simulink model "majorPonepointO1"  (R2023a)
settings: Solver=VariableStepAuto  StartTime=0.0  StopTime=100  RelTol=1e-3
libraries: slpidlib x1
settings Model: Creator=rahul  LastModifiedBy=rahul

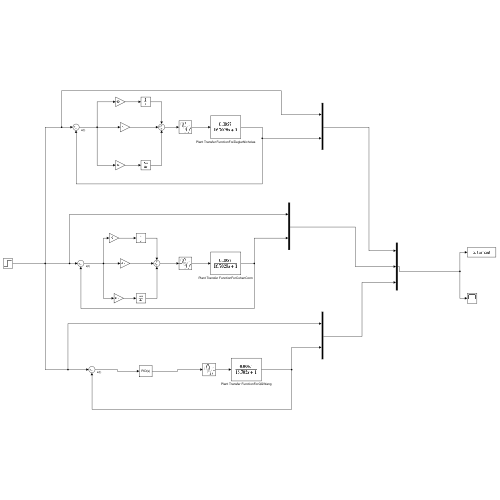
[thumbnail: Simulink's stored preview of the top-level diagram]
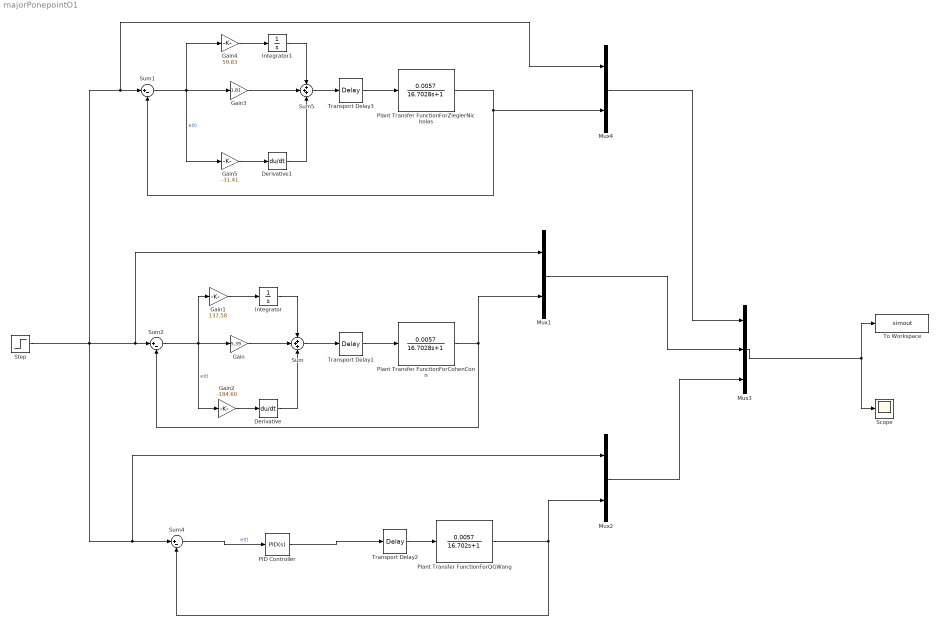
== system majorPonepointO1 ==
  Derivative : Derivative
  Derivative1 : Derivative
  Gain : Gain  Gain=5.39
  Gain1 : Gain  Gain=137.58
  Gain2 : Gain  Gain=-184.60
  Gain3 : Gain  Gain=1.81
  Gain4 : Gain  Gain=59.83
  Gain5 : Gain  Gain=-31.41
  Integrator : Integrator
  Integrator1 : Integrator
  Mux1 : Mux  Inputs=2
  Mux2 : Mux  Inputs=2
  Mux3 : Mux  Inputs=3
  Mux4 : Mux  Inputs=2
  PID Controller : slpidlib/PID Controller  Controller=PID  Form=Parallel  TimeDomain=Continuous-time  UseExternalTs=off  SampleTime=-1  IntegratorMethod=Forward Euler  FilterMethod=Forward Euler  ControllerParametersSource=internal  P=323.18030105094  I=10.7070233456899  UseKiTs=off  D=531.074040829726  N=10.8779684529541  UseFilter=on  TunerSelectOption=Transfer Function Based (PID Tuner App)  InitialConditionSource=internal  InitialConditionForIntegrator=0  InitialConditionForFilter=0  DifferentiatorICPrevScaledInput=0  ExternalReset=none  TrackingMode=off  Kt=1  LimitOutput=off  SatLimitsSource=internal  UpperSaturationLimit=inf  LowerSaturationLimit=-inf  LinearizeAsGain=on  AntiWindupMode=none  Kb=1  LimitIntegrator=off  UpperIntegratorSaturationLimit=inf  LowerIntegratorSaturationLimit=-inf  POutMin=[]  POutMax=[]  IOutMin=[]  IOutMax=[]  DOutMin=[]  DOutMax=[]  NOutMin=[]  NOutMax=[]  SumOutDataTypeStr=double  SumOutMin=[]  SumOutMax=[]  SaturationOutMin=[]  SaturationOutMax=[]  PParamMin=[]  PParamMax=[]  IParamMin=[]  IParamMax=[]  DParamMin=[]  DParamMax=[]  NParamMin=[]  NParamMax=[]  KbParamMin=[]  KbParamMax=[]  KtParamMin=[]  KtParamMax=[]  KbOutMin=[]  KbOutMax=[]  KtOutMin=[]  KtOutMax=[]  IntegratorOutMin=[]  IntegratorOutMax=[]  FilterOutMin=[]  FilterOutMax=[]  SumI1OutMin=[]  SumI1OutMax=[]  SumI2OutMin=[]  SumI2OutMax=[]  SumI3OutMin=[]  SumI3OutMax=[]  SumI4OutMin=[]  SumI4OutMax=[]  SumDOutMin=[]  SumDOutMax=[]  DifferentiatorOutMin=[]  DifferentiatorOutMax=[]  FilterDiffOutCoefMin=[]  FilterDiffOutCoefMax=[]  ReciprocalOutMin=[]  ReciprocalOutMax=[]  SumDenOutMin=[]  SumDenOutMax=[]  SumNumOutMin=[]  SumNumOutMax=[]  DivideOutMin=[]  DivideOutMax=[]  UdiffTsProdOutMin=[]  UdiffTsProdOutMax=[]  NTsProdOutMin=[]  NTsProdOutMax=[]  UintegralTsProdOutMin=[]  UintegralTsProdOutMax=[]  UngainTsProdOutMin=[]  UngainTsProdOutMax=[]  ClampingZeroOutDataTypeStr=Inherit: Inherit via back propagation  ClampingZeroOutMin=[]  ClampingZeroOutMax=[]  FilterDenConstantOutDataTypeStr=Inherit: Inherit via back propagation  FilterDenConstantOutMin=[]  FilterDenConstantOutMax=[]  PCopyOutDataTypeStr=Inherit: Inherit via back propagation  PCopyOutMin=[]  PCopyOutMax=[]  NCopyOutDataTypeStr=Inherit: Inherit via back propagation  NCopyOutMin=[]  NCopyOutMax=[]  IntegratorContinuousStateAttributes=''  IntegratorStateMustResolveToSignalObject=off  IntegratorRTWStateStorageClass=Auto  FilterContinuousStateAttributes=''  FilterStateMustResolveToSignalObject=off  FilterRTWStateStorageClass=Auto  ParallelPVariant=InternalParameters  IdealPVariant=Disabled  IVariant=InternalParameters  DVariant=InternalParameters  IntegratorVariant=Continuous  SatVariant=Disabled  AWVariant=Passthrough  PCopyVariant=Disabled  TRVariant=Disabled  FdbkBlocksVariant=Forward  IdealPFdbkVariant=Disabled  SatFdbkVariant=Disabled  DerivativeFilterVariant=ContFilter  NVariant=InternalParameters  NCopyVariant=Disabled  FilterICVariant=InternalICsFilter  IntegratorICVariant=InternalICs  ExternalResetVariant=Disabled  TRSumVariant=Passthrough  SumFdbkVariant=Disabled  SumVariant=Sum_PID  TsampFilterVariant=InternalTs  TsampNgainVariant=Passthrough  TsampIntegralVariant=Disabled_SignalSpec  ExternalSaturationOutDataTypeStr=Inherit: Same as second input
  Plant Transfer FunctionForCohenConn : TransferFcn  Numerator=[0.0057]  Denominator=[16.7028 1]  ParameterTunability=Optimized
  Plant Transfer FunctionForQGWang : TransferFcn  Numerator=[0.0057]  Denominator=[16.702 1]  ParameterTunability=Optimized
  Plant Transfer FunctionForZieglerNicholas : TransferFcn  Numerator=[0.0057]  Denominator=[16.7028 1]  ParameterTunability=Optimized
  Scope : Scope
  Step : Step  SampleTime=0
  Sum : Sum  Inputs=+++
  Sum1 : Sum  Inputs=|+-
  Sum2 : Sum  Inputs=|+-
  Sum4 : Sum  Inputs=|+-
  Sum5 : Sum  Inputs=+++
  To Workspace : ToWorkspace  VariableName=simout  SaveFormat=Timeseries  SampleTime=-1
  Transport Delay1 : TransportDelay  DelayTime=9.4132
  Transport Delay2 : TransportDelay  DelayTime=9.413
  Transport Delay3 : TransportDelay  DelayTime=9.4132
  wires:
  Plant Transfer FunctionForCohenConn/1 -> Sum2/2, Mux1/2
  Transport Delay1/1 -> Plant Transfer FunctionForCohenConn/1
  Plant Transfer FunctionForQGWang/1 -> Sum4/2, Mux2/2
  Transport Delay2/1 -> Plant Transfer FunctionForQGWang/1
  Mux2/1 -> Mux3/3
  Mux1/1 -> Mux3/2
  Mux3/1 -> Scope/1, To Workspace/1
  Mux4/1 -> Mux3/1
  Transport Delay3/1 -> Plant Transfer FunctionForZieglerNicholas/1
  Plant Transfer FunctionForZieglerNicholas/1 -> Mux4/2, Sum1/2
  Step/1 -> Sum4/1, Mux2/1, Mux4/1, Sum1/1, Mux1/1, Sum2/1
  Sum2/1 -> Gain2/1, Gain/1, Gain1/1  "e(t)"
  Gain1/1 -> Integrator/1
  Gain/1 -> Sum/2
  Sum/1 -> Transport Delay1/1
  Gain2/1 -> Derivative/1
  Integrator/1 -> Sum/1
  Derivative/1 -> Sum/3
  Derivative1/1 -> Sum5/3
  Gain5/1 -> Derivative1/1
  Gain3/1 -> Sum5/2
  Integrator1/1 -> Sum5/1
  Sum1/1 -> Gain3/1, Gain5/1, Gain4/1  "e(t)"
  Gain4/1 -> Integrator1/1
  Sum5/1 -> Transport Delay3/1
  Sum4/1 -> PID Controller/1  "e(t)"
  PID Controller/1 -> Transport Delay2/1
